simulink model "quadcopter_hadi"  (R2020a)
settings: Solver=FixedStepAuto  StartTime=0.0  StopTime=options.T_train  FixedStep=options.dt  RelTol=1e-3
undefined symbols (not defined in the file or in its folder): options
libraries: neural x134, simulink x3
(part 2 of 6)

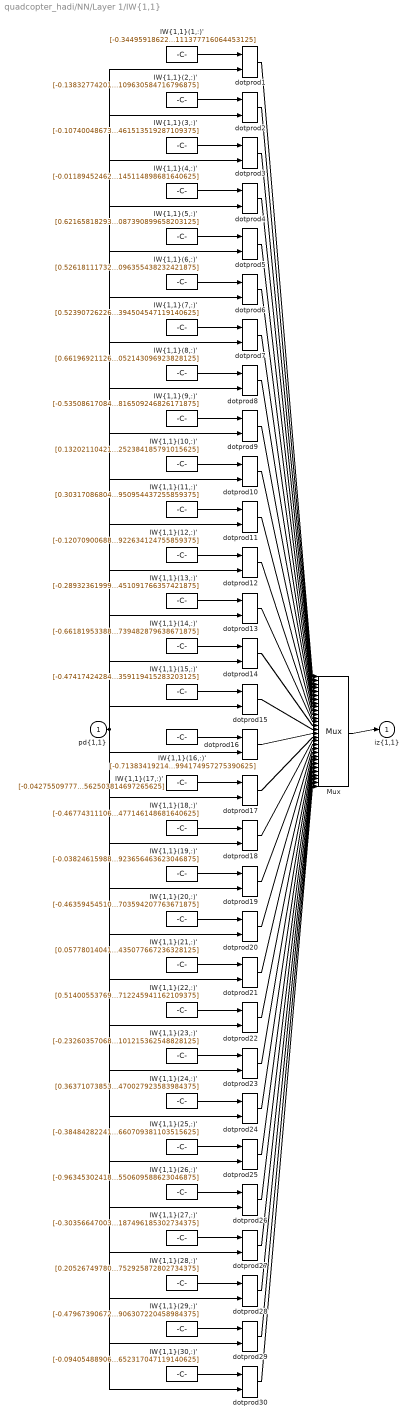
== system quadcopter_hadi/NN/Layer 1/IW{1,1} ==
  "pd{1,1}" : Inport  PortDimensions=12
      mask Display: e = 0.06;c1 = [120 230 180]/255;c2 = ([120 230 180]+0)/(256+128);c3 = ([120 230 180]+128)/(256+128);patch([0 1 1 0],[0 0 1 1],c1);patch([0 1 1 1-e 1-e 0+e],[0 0 1 1-e 0+e 0+e],c2);patch([0 0 1 1-e 0+e 0+e],[0 1 1 1-e 1-e 0+e],c3);plot([0 1 1 0 0],[0 0 1 1 0]);
  "IW{1,1}(1,:)'" : Constant  Value=[-0.34495918622896504235342263200436718761920928955078125;-0.337043723826467189752520425827242434024810791015625;-0.353509203138535899046956956226495094597339630126953125;-0.203038619812965226429923859541304409503936767578125;0.6070294560030344843681859856587834656238555908203125;-0.53053426435416162210145785138593055307865142822265625;0.40549662019742005458766698211547918617725372314453125;-0.57742825274382714173526665035751648247241973876953125;-0.318931166570593116471599159922334365546703338623046875;0.062207561993730724203555126905484939925372600555419921875;0.340697979277285567523136933232308365404605865478515625;-0.4455201013994714021038134887930937111377716064453125]
      mask Display: e = 0.06;c1 = [120 150 230]/255;c2 = ([120 150 230]+0)/383;c3 = ([120 150 230]+128)/383;patch([0 1 1 0],[0 0 1 1],c1);patch([0 1 1 1-e 1-e 0+e],[0 0 1 1-e 0+e 0+e],c2);patch([0 0 1 1-e 0+e 0+e],[0 1 1 1-e 1-e 0+e],c3);plot([0 1 1 0 0],[0 0 1 1 0]);disp('Weights');
  "IW{1,1}(10,:)'" : Constant  Value=[0.1320211042100700726820150521234609186649322509765625;-0.668627746850793958088843282894231379032135009765625;0.5677864448354277282504654067452065646648406982421875;0.0876991445872624397761541104046045802533626556396484375;-0.56179042828860958902481570476084016263484954833984375;-0.348882703813149508409452437263098545372486114501953125;0.20436817069308166328056586280581541359424591064453125;0.52533055189570043719271552618010900914669036865234375;0.9640955257051808668933290391578339040279388427734375;0.24519760024947567789155300488346256315708160400390625;-0.54886720284928236512911325917229987680912017822265625;0.257390461906887024756684922977001406252384185791015625]
      mask Display: e = 0.06;c1 = [120 150 230]/255;c2 = ([120 150 230]+0)/383;c3 = ([120 150 230]+128)/383;patch([0 1 1 0],[0 0 1 1],c1);patch([0 1 1 1-e 1-e 0+e],[0 0 1 1-e 0+e 0+e],c2);patch([0 0 1 1-e 0+e 0+e],[0 1 1 1-e 1-e 0+e],c3);plot([0 1 1 0 0],[0 0 1 1 0]);disp('Weights');
  "IW{1,1}(11,:)'" : Constant  Value=[0.303170868046250541194552852175547741353511810302734375;0.417696798526436541276751768236863426864147186279296875;0.298261926050533421328481153977918438613414764404296875;0.255036537942097740749858303388464264571666717529296875;-0.7244894696039654302666122021037153899669647216796875;0.384577235401244943435727918767952360212802886962890625;0.50089881261622692942836465590517036616802215576171875;0.309950678139630564356110653534415178000926971435546875;-0.237501763203682936254068636117153801023960113525390625;0.352274481786692350571144061177619732916355133056640625;0.416167732301852222320803775801323354244232177734375;0.319139822380907600685162606168887577950954437255859375]
      mask Display: e = 0.06;c1 = [120 150 230]/255;c2 = ([120 150 230]+0)/383;c3 = ([120 150 230]+128)/383;patch([0 1 1 0],[0 0 1 1],c1);patch([0 1 1 1-e 1-e 0+e],[0 0 1 1-e 0+e 0+e],c2);patch([0 0 1 1-e 0+e 0+e],[0 1 1 1-e 1-e 0+e],c3);plot([0 1 1 0 0],[0 0 1 1 0]);disp('Weights');
  "IW{1,1}(12,:)'" : Constant  Value=[-0.12070900688584484949927855268470011651515960693359375;0.53505476241080895949409068634849973022937774658203125;-0.2381029444773878067653782863999367691576480865478515625;-0.5429788112757945039987816926441155374050140380859375;-0.63257154591633291129681992970290593802928924560546875;-0.661157862985402022815151212853379547595977783203125;-0.60701795231436894706433804458356462419033050537109375;-0.1298953163042863290232986628325306810438632965087890625;0.84804820628712374031010767794214189052581787109375;0.126838248292744426581890593297430314123630523681640625;-0.1101413285813153120074048274545930325984954833984375;0.29384196869861722856143160242936573922634124755859375]
      mask Display: e = 0.06;c1 = [120 150 230]/255;c2 = ([120 150 230]+0)/383;c3 = ([120 150 230]+128)/383;patch([0 1 1 0],[0 0 1 1],c1);patch([0 1 1 1-e 1-e 0+e],[0 0 1 1-e 0+e 0+e],c2);patch([0 0 1 1-e 0+e 0+e],[0 1 1 1-e 1-e 0+e],c3);plot([0 1 1 0 0],[0 0 1 1 0]);disp('Weights');
  "IW{1,1}(13,:)'" : Constant  Value=[-0.289323619993917702242214318175683729350566864013671875;-0.5661963662077675873973703346564434468746185302734375;-0.263001047924680708689493258134461939334869384765625;0.763890200972800581524779772735200822353363037109375;0.58754737292300973638958794253994710743427276611328125;0.60801383959154453595630229756352491676807403564453125;-0.5265003431597750083170694779255427420139312744140625;0.1137610485372035629136888701395946554839611053466796875;-0.5072867886078873400634847712353803217411041259765625;0.469464342242350340939083253033459186553955078125;0.277240104279838639467214989053900353610515594482421875;-0.793994998950516173152891497011296451091766357421875]
      mask Display: e = 0.06;c1 = [120 150 230]/255;c2 = ([120 150 230]+0)/383;c3 = ([120 150 230]+128)/383;patch([0 1 1 0],[0 0 1 1],c1);patch([0 1 1 1-e 1-e 0+e],[0 0 1 1-e 0+e 0+e],c2);patch([0 0 1 1-e 0+e 0+e],[0 1 1 1-e 1-e 0+e],c3);plot([0 1 1 0 0],[0 0 1 1 0]);disp('Weights');
  "IW{1,1}(14,:)'" : Constant  Value=[-0.66181953388010417160813858572510071098804473876953125;-0.0703899958783368584480655272272997535765171051025390625;-0.5991581448220273387050838209688663482666015625;0.3699087288651252691806803341023623943328857421875;-0.317569978247375761526427595526911318302154541015625;0.52610263318384575814690151673858053982257843017578125;-0.27980528750779820601479741526418365538120269775390625;0.416857080760284326448328329206560738384723663330078125;0.725583975883678622409433955908752977848052978515625;0.435054608829613831399996115578687749803066253662109375;-0.458054194167220318778532828218885697424411773681640625;-0.69641998097306412329743352529476396739482879638671875]
      mask Display: e = 0.06;c1 = [120 150 230]/255;c2 = ([120 150 230]+0)/383;c3 = ([120 150 230]+128)/383;patch([0 1 1 0],[0 0 1 1],c1);patch([0 1 1 1-e 1-e 0+e],[0 0 1 1-e 0+e 0+e],c2);patch([0 0 1 1-e 0+e 0+e],[0 1 1 1-e 1-e 0+e],c3);plot([0 1 1 0 0],[0 0 1 1 0]);disp('Weights');
  "IW{1,1}(15,:)'" : Constant  Value=[-0.474174242849191351911741776348208077251911163330078125;-0.04891747802004135781128724147492903284728527069091796875;0.411091414463095439213446979920263402163982391357421875;-0.03650572612073470224469673439671169035136699676513671875;0.9444343014165463845444037360721267759799957275390625;0.59688073236543626176597854282590560615062713623046875;0.218856619672374519414148608120740391314029693603515625;0.051222945628977611942644898590515367686748504638671875;-0.53026532302764384230187033608672209084033966064453125;-0.25745047520204378255215260651311837136745452880859375;-0.28207174996604778005604430290986783802509307861328125;-0.69241459640721547685870973509736359119415283203125]
      mask Display: e = 0.06;c1 = [120 150 230]/255;c2 = ([120 150 230]+0)/383;c3 = ([120 150 230]+128)/383;patch([0 1 1 0],[0 0 1 1],c1);patch([0 1 1 1-e 1-e 0+e],[0 0 1 1-e 0+e 0+e],c2);patch([0 0 1 1-e 0+e 0+e],[0 1 1 1-e 1-e 0+e],c3);plot([0 1 1 0 0],[0 0 1 1 0]);disp('Weights');
  "IW{1,1}(16,:)'" : Constant  Value=[-0.7138341921425268576939515696722082793712615966796875;0.037340534291947467815386829670387669466435909271240234375;0.54479666790288738820180469701881520450115203857421875;-0.2021602873810667555520836913274251855909824371337890625;-0.007519167787261805437071249258451643981970846652984619140625;-0.53077415040406428214936340737040154635906219482421875;-0.5226709505181668102835601530387066304683685302734375;0.723058432424417585338005665107630193233489990234375;0.57923937859777441250486162971355952322483062744140625;-0.11337543588273957251288948100409470498561859130859375;0.401730100819205071527306927237077616155147552490234375;-0.468101990603508932853316082400851882994174957275390625]
      mask Display: e = 0.06;c1 = [120 150 230]/255;c2 = ([120 150 230]+0)/383;c3 = ([120 150 230]+128)/383;patch([0 1 1 0],[0 0 1 1],c1);patch([0 1 1 1-e 1-e 0+e],[0 0 1 1-e 0+e 0+e],c2);patch([0 0 1 1-e 0+e 0+e],[0 1 1 1-e 1-e 0+e],c3);plot([0 1 1 0 0],[0 0 1 1 0]);disp('Weights');
  "IW{1,1}(17,:)'" : Constant  Value=[-0.042755097773684337669752864030670025385916233062744140625;0.756605493708306209299507827381603419780731201171875;-0.49321543387669442015663889833376742899417877197265625;-0.325875695135673992819391742159496061503887176513671875;0.74621132739286133439549075774266384541988372802734375;-0.08679338092441117591402388597998651675879955291748046875;-0.453659556696276944354195848063682205975055694580078125;-0.62366920735145792153986121775233186781406402587890625;-0.8150300553565761330077066304511390626430511474609375;0.11508615117670083216605547704602940939366817474365234375;0.50080307025032577694645397059503011405467987060546875;-0.1889869390507021851277613677666522562503814697265625]
      mask Display: e = 0.06;c1 = [120 150 230]/255;c2 = ([120 150 230]+0)/383;c3 = ([120 150 230]+128)/383;patch([0 1 1 0],[0 0 1 1],c1);patch([0 1 1 1-e 1-e 0+e],[0 0 1 1-e 0+e 0+e],c2);patch([0 0 1 1-e 0+e 0+e],[0 1 1 1-e 1-e 0+e],c3);plot([0 1 1 0 0],[0 0 1 1 0]);disp('Weights');
  "IW{1,1}(18,:)'" : Constant  Value=[-0.46774311106672594728905778538319282233715057373046875;0.6841256626066598567348364667850546538829803466796875;0.9849894355797144118724872896564193069934844970703125;-0.68550119697938216578592118821688927710056304931640625;0.330176687462999274291775009260163642466068267822265625;-0.0757421832731329514043494555153301917016506195068359375;-0.447741975939116854110721988035948015749454498291015625;0.39313879995946365841774650107254274189472198486328125;0.039471528533331634580605395967722870409488677978515625;0.02006562823856268551470094507749308831989765167236328125;-0.39311485574848881174858661324833519756793975830078125;-0.0087918173201730898114192314096726477146148681640625]
      mask Display: e = 0.06;c1 = [120 150 230]/255;c2 = ([120 150 230]+0)/383;c3 = ([120 150 230]+128)/383;patch([0 1 1 0],[0 0 1 1],c1);patch([0 1 1 1-e 1-e 0+e],[0 0 1 1-e 0+e 0+e],c2);patch([0 0 1 1-e 0+e 0+e],[0 1 1 1-e 1-e 0+e],c3);plot([0 1 1 0 0],[0 0 1 1 0]);disp('Weights');
  "IW{1,1}(19,:)'" : Constant  Value=[-0.038246159880512074769054464695727801881730556488037109375;-0.352676020543882307034522227695561014115810394287109375;0.55521428620525714592304211691953241825103759765625;-0.236763462408719538299095574984676204621791839599609375;-0.072727039559656869727177763707004487514495849609375;0.121413069532788242543830392605741508305072784423828125;-0.305176260105177010739652132542687468230724334716796875;-0.4439076777797945627668241286301054060459136962890625;-0.98313794595444570223463642832939513027667999267578125;-0.1270463796308993476014137513629975728690624237060546875;0.902189168883986258862250906531699001789093017578125;-0.1273899410450269609196283226992818526923656463623046875]
      mask Display: e = 0.06;c1 = [120 150 230]/255;c2 = ([120 150 230]+0)/383;c3 = ([120 150 230]+128)/383;patch([0 1 1 0],[0 0 1 1],c1);patch([0 1 1 1-e 1-e 0+e],[0 0 1 1-e 0+e 0+e],c2);patch([0 0 1 1-e 0+e 0+e],[0 1 1 1-e 1-e 0+e],c3);plot([0 1 1 0 0],[0 0 1 1 0]);disp('Weights');
  "IW{1,1}(2,:)'" : Constant  Value=[-0.138327742010193599497824834543280303478240966796875;-0.8821579573578286481705390542629174888134002685546875;-0.086774823339577478176209979210398159921169281005859375;0.574481836593661920886688676546327769756317138671875;-0.529761642169075397390543002984486520290374755859375;-0.10542287766760018163925138878767029382288455963134765625;-0.439906734367202567614896224768017418682575225830078125;-0.2072733028239615304944010176768642850220203399658203125;0.56108927501055705366894699182012118399143218994140625;-0.59696070904831877168561504731769673526287078857421875;0.363071184175628058898865901937824673950672149658203125;0.826574201384250084601035268860869109630584716796875]
      mask Display: e = 0.06;c1 = [120 150 230]/255;c2 = ([120 150 230]+0)/383;c3 = ([120 150 230]+128)/383;patch([0 1 1 0],[0 0 1 1],c1);patch([0 1 1 1-e 1-e 0+e],[0 0 1 1-e 0+e 0+e],c2);patch([0 0 1 1-e 0+e 0+e],[0 1 1 1-e 1-e 0+e],c3);plot([0 1 1 0 0],[0 0 1 1 0]);disp('Weights');
  "IW{1,1}(20,:)'" : Constant  Value=[-0.463594545102451238705043579102493822574615478515625;0.59859312767452277359581103155505843460559844970703125;0.60801387674530882332391001909854821860790252685546875;-0.4376213200013177040403888895525597035884857177734375;0.465343080687624366387211694018333218991756439208984375;-0.7504994595920637667774144574650563299655914306640625;0.1096976721316818281781735322510940022766590118408203125;0.73737837988444632220108587716822512447834014892578125;-0.4011595462138346501745900241076014935970306396484375;-0.4637681719671171709507007108186371624469757080078125;-0.449027218825725438211549089828622527420520782470703125;0.1021728787905504531874356644038925878703594207763671875]
      mask Display: e = 0.06;c1 = [120 150 230]/255;c2 = ([120 150 230]+0)/383;c3 = ([120 150 230]+128)/383;patch([0 1 1 0],[0 0 1 1],c1);patch([0 1 1 1-e 1-e 0+e],[0 0 1 1-e 0+e 0+e],c2);patch([0 0 1 1-e 0+e 0+e],[0 1 1 1-e 1-e 0+e],c3);plot([0 1 1 0 0],[0 0 1 1 0]);disp('Weights');
  "IW{1,1}(21,:)'" : Constant  Value=[0.057780140416524870816683545626801787875592708587646484375;0.3446971110697958362578674496035091578960418701171875;0.449399367813893835243987950889277271926403045654296875;-0.443821935475689155481404668535105884075164794921875;-0.6004000148789756519107640997390262782573699951171875;0.5221656918855515083777163454215042293071746826171875;0.7545170196760597747243082267232239246368408203125;0.6769434357346761910179111509933136403560638427734375;-0.354202449623008230883414171330514363944530487060546875;-0.6879409685100552618308711316785775125026702880859375;-0.47037002086478107987232988307368941605091094970703125;-0.036409196162681962960494530534560908563435077667236328125]
      mask Display: e = 0.06;c1 = [120 150 230]/255;c2 = ([120 150 230]+0)/383;c3 = ([120 150 230]+128)/383;patch([0 1 1 0],[0 0 1 1],c1);patch([0 1 1 1-e 1-e 0+e],[0 0 1 1-e 0+e 0+e],c2);patch([0 0 1 1-e 0+e 0+e],[0 1 1 1-e 1-e 0+e],c3);plot([0 1 1 0 0],[0 0 1 1 0]);disp('Weights');
  "IW{1,1}(22,:)'" : Constant  Value=[0.5140055376953736043788012466393411159515380859375;-0.5947686065042745440223370678722858428955078125;0.5873305202085770115871810048702172935009002685546875;-0.3123825429203936909772210128721781075000762939453125;0.53040919266754682492859274134389124810695648193359375;-0.512060005984212640584019027301110327243804931640625;-0.58357904592260589904384460169239901006221771240234375;-0.65324640661213795311823560041375458240509033203125;0.11144911224205389377317487742402590811252593994140625;0.518976412161789912858012030483223497867584228515625;0.444696308915158267094369648475549183785915374755859375;0.37402510131684285621389562948024831712245941162109375]
      mask Display: e = 0.06;c1 = [120 150 230]/255;c2 = ([120 150 230]+0)/383;c3 = ([120 150 230]+128)/383;patch([0 1 1 0],[0 0 1 1],c1);patch([0 1 1 1-e 1-e 0+e],[0 0 1 1-e 0+e 0+e],c2);patch([0 0 1 1-e 0+e 0+e],[0 1 1 1-e 1-e 0+e],c3);plot([0 1 1 0 0],[0 0 1 1 0]);disp('Weights');
  "IW{1,1}(23,:)'" : Constant  Value=[-0.232603570682247184908675308179226703941822052001953125;1.0517575952902709079950227533117868006229400634765625;0.192098506547794423138242336790426634252071380615234375;-0.32973101267621285348496940059703774750232696533203125;-0.11914062282579916673963538187308586202561855316162109375;-0.382401536887546911192004017721046693623065948486328125;-0.35312961938715103915598092498839832842350006103515625;0.164251234547107827221879006174276582896709442138671875;0.407895691716687769368121507795876823365688323974609375;-0.8752379671019092644002057568286545574665069580078125;0.413170407813726325851888532270095311105251312255859375;0.61017749365807916195336702003260143101215362548828125]
      mask Display: e = 0.06;c1 = [120 150 230]/255;c2 = ([120 150 230]+0)/383;c3 = ([120 150 230]+128)/383;patch([0 1 1 0],[0 0 1 1],c1);patch([0 1 1 1-e 1-e 0+e],[0 0 1 1-e 0+e 0+e],c2);patch([0 0 1 1-e 0+e 0+e],[0 1 1 1-e 1-e 0+e],c3);plot([0 1 1 0 0],[0 0 1 1 0]);disp('Weights');
  "IW{1,1}(24,:)'" : Constant  Value=[0.363710738539707645333720620328676886856555938720703125;-0.09612229443336224588012584035823238082230091094970703125;0.1808198562023227429218508177655166946351528167724609375;-0.4720334048143357552618226691265590488910675048828125;-0.294063177509011897114987732493318617343902587890625;0.87626234603710873027893057951587252318859100341796875;-0.634035117918139601300708818598650395870208740234375;-0.5522125975537324205077993610757403075695037841796875;-0.17623578995034094862859319619019515812397003173828125;0.43632440477811285095555149382562376558780670166015625;0.89163382673504631981131751672364771366119384765625;-0.167074453475141326830311072626500390470027923583984375]
      mask Display: e = 0.06;c1 = [120 150 230]/255;c2 = ([120 150 230]+0)/383;c3 = ([120 150 230]+128)/383;patch([0 1 1 0],[0 0 1 1],c1);patch([0 1 1 1-e 1-e 0+e],[0 0 1 1-e 0+e 0+e],c2);patch([0 0 1 1-e 0+e 0+e],[0 1 1 1-e 1-e 0+e],c3);plot([0 1 1 0 0],[0 0 1 1 0]);disp('Weights');
  "IW{1,1}(25,:)'" : Constant  Value=[-0.38484282241698941628982311158324591815471649169921875;0.209383083397630065380923269913182593882083892822265625;-0.6135781360303920184406933913123793900012969970703125;0.76016324948769209424170867350767366588115692138671875;-0.362471393437067190834710572744370438158512115478515625;-0.60581492990217078453696331052924506366252899169921875;0.585753156661642293556724325753748416900634765625;-0.50309249495567087695491181875695474445819854736328125;0.48695535648605725587145798272104002535343170166015625;0.714144675850457932853032616549171507358551025390625;-0.27025145430345942632044398123980499804019927978515625;0.541591787927542700487038018763996660709381103515625]
      mask Display: e = 0.06;c1 = [120 150 230]/255;c2 = ([120 150 230]+0)/383;c3 = ([120 150 230]+128)/383;patch([0 1 1 0],[0 0 1 1],c1);patch([0 1 1 1-e 1-e 0+e],[0 0 1 1-e 0+e 0+e],c2);patch([0 0 1 1-e 0+e 0+e],[0 1 1 1-e 1-e 0+e],c3);plot([0 1 1 0 0],[0 0 1 1 0]);disp('Weights');
  "IW{1,1}(26,:)'" : Constant  Value=[-0.96345302418685896395089685029233805835247039794921875;0.2905057488862652359529192835907451808452606201171875;0.25145319652790931730379497821559198200702667236328125;-0.110023152779389732369708099213312380015850067138671875;0.80159591366269555834378479630686342716217041015625;0.62482096118850416477386033875518478453159332275390625;0.1804782462712755941591780128874233923852443695068359375;-0.69123516144817764850216690319939516484737396240234375;-0.32694257387283298665892061762860976159572601318359375;0.04918257558373796689554779959507868625223636627197265625;-0.66886565497689642878498261779895983636379241943359375;-0.27607850951602752598290635432931594550609588623046875]
      mask Display: e = 0.06;c1 = [120 150 230]/255;c2 = ([120 150 230]+0)/383;c3 = ([120 150 230]+128)/383;patch([0 1 1 0],[0 0 1 1],c1);patch([0 1 1 1-e 1-e 0+e],[0 0 1 1-e 0+e 0+e],c2);patch([0 0 1 1-e 0+e 0+e],[0 1 1 1-e 1-e 0+e],c3);plot([0 1 1 0 0],[0 0 1 1 0]);disp('Weights');
  "IW{1,1}(27,:)'" : Constant  Value=[-0.30356647003768255643763041007332503795623779296875;0.397535672113617177814148817560635507106781005859375;-0.12467461340805656433428083573744515888392925262451171875;-0.70752774859209655033964736503548920154571533203125;0.66465656668955952479649340602918528020381927490234375;-0.034394405255799960496876366278229397721588611602783203125;0.48028770547293431203428326625726185739040374755859375;-0.54949688236805938057472076252452097833156585693359375;-0.81716499127206809749424110123072750866413116455078125;-0.00698809762742241304123158585070996196009218692779541015625;0.66303543817856114284126078928238712251186370849609375;0.126087445960947286405229306183173321187496185302734375]
      mask Display: e = 0.06;c1 = [120 150 230]/255;c2 = ([120 150 230]+0)/383;c3 = ([120 150 230]+128)/383;patch([0 1 1 0],[0 0 1 1],c1);patch([0 1 1 1-e 1-e 0+e],[0 0 1 1-e 0+e 0+e],c2);patch([0 0 1 1-e 0+e 0+e],[0 1 1 1-e 1-e 0+e],c3);plot([0 1 1 0 0],[0 0 1 1 0]);disp('Weights');
  "IW{1,1}(28,:)'" : Constant  Value=[0.2052674978043443621000818666288978420197963714599609375;0.35070641269276559004453019952052272856235504150390625;0.63836983163101723715016078131156973540782928466796875;0.391881550618063290158943345886655151844024658203125;-0.171565904611522268563561510745785199105739593505859375;-0.54250734055331950589362577375140972435474395751953125;-0.70606196712206215071461201659985817968845367431640625;0.315078701273152239625829906799481250345706939697265625;0.7571027888427377394719997028005309402942657470703125;0.374860392792828178709640951637993566691875457763671875;-0.2434391219306188958171333069913089275360107421875;0.44060900182772877453629689625813625752925872802734375]
      mask Display: e = 0.06;c1 = [120 150 230]/255;c2 = ([120 150 230]+0)/383;c3 = ([120 150 230]+128)/383;patch([0 1 1 0],[0 0 1 1],c1);patch([0 1 1 1-e 1-e 0+e],[0 0 1 1-e 0+e 0+e],c2);patch([0 0 1 1-e 0+e 0+e],[0 1 1 1-e 1-e 0+e],c3);plot([0 1 1 0 0],[0 0 1 1 0]);disp('Weights');
  "IW{1,1}(29,:)'" : Constant  Value=[-0.47967390672573750887153209987445734441280364990234375;-0.1710937102409248178336298451540642417967319488525390625;0.51569510317060884840856260780128650367259979248046875;0.58303215536935770746396201502648182213306427001953125;0.5397101537550013095057011014432646334171295166015625;0.491815641277797033215080091395066119730472564697265625;-0.26359399694002305647444472924689762294292449951171875;-0.5159654272192575330535646571661345660686492919921875;-0.795397536289371931417235828121192753314971923828125;-0.67850322234585813685470156997325830161571502685546875;0.394304169753736000192390065421932376921176910400390625;0.08171990282033135544192958832354634068906307220458984375]
      mask Display: e = 0.06;c1 = [120 150 230]/255;c2 = ([120 150 230]+0)/383;c3 = ([120 150 230]+128)/383;patch([0 1 1 0],[0 0 1 1],c1);patch([0 1 1 1-e 1-e 0+e],[0 0 1 1-e 0+e 0+e],c2);patch([0 0 1 1-e 0+e 0+e],[0 1 1 1-e 1-e 0+e],c3);plot([0 1 1 0 0],[0 0 1 1 0]);disp('Weights');
  "IW{1,1}(3,:)'" : Constant  Value=[-0.10740048673439391013761934345893678255379199981689453125;-0.2172720702613431253968911960328114219009876251220703125;0.2378394016623203988114454432434285990893840789794921875;0.51394110379334267957318616026896052062511444091796875;0.37661624669478188653926054030307568609714508056640625;0.487273539589460569221301966535975225269794464111328125;0.42566721914787331026985839343979023396968841552734375;-0.8937639297673716232139895510044880211353302001953125;-0.135569594033347284867119242335320450365543365478515625;0.8757068982107643062562374325352720916271209716796875;0.361943270803529892898353637065156362950801849365234375;-0.135562992761426581722616901970468461513519287109375]
      mask Display: e = 0.06;c1 = [120 150 230]/255;c2 = ([120 150 230]+0)/383;c3 = ([120 150 230]+128)/383;patch([0 1 1 0],[0 0 1 1],c1);patch([0 1 1 1-e 1-e 0+e],[0 0 1 1-e 0+e 0+e],c2);patch([0 0 1 1-e 0+e 0+e],[0 1 1 1-e 1-e 0+e],c3);plot([0 1 1 0 0],[0 0 1 1 0]);disp('Weights');
  "IW{1,1}(30,:)'" : Constant  Value=[-0.09405488906321969599932941719089285470545291900634765625;-0.467610333580071202419503606506623327732086181640625;-0.159695215182861172120709625232848338782787322998046875;0.322947655372797848283283883574767969548702239990234375;0.337291546166701483588923338174936361610889434814453125;-0.5604847262703398502736718000960536301136016845703125;-0.51864010655251202575044544573756866157054901123046875;0.55916502354967179133637955601443536579608917236328125;-0.379802758147711305714011587042477913200855255126953125;0.91760468236122061380655168250086717307567596435546875;-0.04817922357743227579351952272190828807651996612548828125;-0.79844520344081149065829094979562796652317047119140625]
      mask Display: e = 0.06;c1 = [120 150 230]/255;c2 = ([120 150 230]+0)/383;c3 = ([120 150 230]+128)/383;patch([0 1 1 0],[0 0 1 1],c1);patch([0 1 1 1-e 1-e 0+e],[0 0 1 1-e 0+e 0+e],c2);patch([0 0 1 1-e 0+e 0+e],[0 1 1 1-e 1-e 0+e],c3);plot([0 1 1 0 0],[0 0 1 1 0]);disp('Weights');
  "IW{1,1}(4,:)'" : Constant  Value=[-0.01189452462799470318366434895551719819195568561553955078125;0.30955222784386149381674613323411904275417327880859375;0.37405694379270337801557388957007788121700286865234375;-0.337930186454908021431720044347457587718963623046875;0.5586613099046164876426701084710657596588134765625;0.66911143805661854599975413293577730655670166015625;-0.71804193868486254626049003491061739623546600341796875;-0.30199328076909093265811634410056285560131072998046875;0.479407886897864343733743908160249702632427215576171875;-0.2214060732027794686782584676620899699628353118896484375;-0.52388837611547189876404218011884950101375579833984375;0.9040601619831820645600828356691636145114898681640625]
      mask Display: e = 0.06;c1 = [120 150 230]/255;c2 = ([120 150 230]+0)/383;c3 = ([120 150 230]+128)/383;patch([0 1 1 0],[0 0 1 1],c1);patch([0 1 1 1-e 1-e 0+e],[0 0 1 1-e 0+e 0+e],c2);patch([0 0 1 1-e 0+e 0+e],[0 1 1 1-e 1-e 0+e],c3);plot([0 1 1 0 0],[0 0 1 1 0]);disp('Weights');
  "IW{1,1}(5,:)'" : Constant  Value=[0.62165818293616614820251697892672382295131683349609375;0.397865582455294575225934750051237642765045166015625;0.7316722067555614383849160731188021600246429443359375;-0.487716561673313453439959630486555397510528564453125;-0.30403759874493208048562564727035351097583770751953125;0.36844925044632315103143582746270112693309783935546875;-0.2266763489839582756957270248676650226116180419921875;-0.332136918694305782739917276558117009699344635009765625;0.1219087873483228889881502254866063594818115234375;0.48112981175821623036625851455028168857097625732421875;0.3560647281492952398451734552509151399135589599609375;0.55496834794659843925757058968883939087390899658203125]
      mask Display: e = 0.06;c1 = [120 150 230]/255;c2 = ([120 150 230]+0)/383;c3 = ([120 150 230]+128)/383;patch([0 1 1 0],[0 0 1 1],c1);patch([0 1 1 1-e 1-e 0+e],[0 0 1 1-e 0+e 0+e],c2);patch([0 0 1 1-e 0+e 0+e],[0 1 1 1-e 1-e 0+e],c3);plot([0 1 1 0 0],[0 0 1 1 0]);disp('Weights');
  "IW{1,1}(6,:)'" : Constant  Value=[0.52618111732526784418695342537830583751201629638671875;-0.440625471004194635415984748760820366442203521728515625;-0.62487389944786653206421078721177764236927032470703125;-0.0222850483937825256941511753439044696278870105743408203125;0.5691934711227240040187780323321931064128875732421875;-0.90291982242941315472961605337332002818584442138671875;0.417050626719000394615477489423938095569610595703125;-0.177028368010524517206505379363079555332660675048828125;-0.15451508861587426313377591213793493807315826416015625;0.75850356023963472207327640717267058789730072021484375;-0.195424851993045878284505079136579297482967376708984375;0.1381647165547894295922759511086042039096355438232421875]
      mask Display: e = 0.06;c1 = [120 150 230]/255;c2 = ([120 150 230]+0)/383;c3 = ([120 150 230]+128)/383;patch([0 1 1 0],[0 0 1 1],c1);patch([0 1 1 1-e 1-e 0+e],[0 0 1 1-e 0+e 0+e],c2);patch([0 0 1 1-e 0+e 0+e],[0 1 1 1-e 1-e 0+e],c3);plot([0 1 1 0 0],[0 0 1 1 0]);disp('Weights');
  "IW{1,1}(7,:)'" : Constant  Value=[0.5239072622656049116329768366995267570018768310546875;-0.3432914261529236288339461680152453482151031494140625;-0.7086167696794871684318195548257790505886077880859375;0.5572090256839017374801414916873909533023834228515625;-0.56712716940789198449834884740994311869144439697265625;0.061168833619787581212801086394392768852412700653076171875;-0.643665616440932009112430023378692567348480224609375;-0.38315560147590821404861571863875724375247955322265625;0.52732661808370517864119619844132103025913238525390625;0.4970608747190905507551406117272563278675079345703125;0.224618568925987471818217500185710377991199493408203125;-0.344126400018276046299803283545770682394504547119140625]
      mask Display: e = 0.06;c1 = [120 150 230]/255;c2 = ([120 150 230]+0)/383;c3 = ([120 150 230]+128)/383;patch([0 1 1 0],[0 0 1 1],c1);patch([0 1 1 1-e 1-e 0+e],[0 0 1 1-e 0+e 0+e],c2);patch([0 0 1 1-e 0+e 0+e],[0 1 1 1-e 1-e 0+e],c3);plot([0 1 1 0 0],[0 0 1 1 0]);disp('Weights');
  "IW{1,1}(8,:)'" : Constant  Value=[0.661969211261337786567082730471156537532806396484375;-0.0383159852429298675158264586571021936833858489990234375;-0.09722917799189277621163540743509656749665737152099609375;0.2607808122246872972738174212281592190265655517578125;-0.89249206258839197669630038944887928664684295654296875;0.290074660908613335408290367922745645046234130859375;0.082028400526420741645239331774064339697360992431640625;0.52493892311090950553165157543844543397426605224609375;0.76704115696658570211496908086701296269893646240234375;-0.240414255138845456283291923682554624974727630615234375;-0.023871623658473208051677971752724261023104190826416015625;-0.63902701740953304909709231651504524052143096923828125]
      mask Display: e = 0.06;c1 = [120 150 230]/255;c2 = ([120 150 230]+0)/383;c3 = ([120 150 230]+128)/383;patch([0 1 1 0],[0 0 1 1],c1);patch([0 1 1 1-e 1-e 0+e],[0 0 1 1-e 0+e 0+e],c2);patch([0 0 1 1-e 0+e 0+e],[0 1 1 1-e 1-e 0+e],c3);plot([0 1 1 0 0],[0 0 1 1 0]);disp('Weights');
  "IW{1,1}(9,:)'" : Constant  Value=[-0.53508617084060328128458650098764337599277496337890625;0.0795815485999021021701338440834661014378070831298828125;-0.66131439300399819103404297493398189544677734375;0.198887915850595120570432072781841270625591278076171875;-0.4638113422795602236448075927910394966602325439453125;-0.5485711737735516901892651731031946837902069091796875;0.39899541815562844515596907513099722564220428466796875;-0.017703826639693880096171341165245394222438335418701171875;0.91695552187400952703910661512054502964019775390625;-0.148963777410568931625078903380199335515499114990234375;-0.43559264363035443690108650116599164903163909912109375;-0.27085804944175506658865515419165603816509246826171875]
      mask Display: e = 0.06;c1 = [120 150 230]/255;c2 = ([120 150 230]+0)/383;c3 = ([120 150 230]+128)/383;patch([0 1 1 0],[0 0 1 1],c1);patch([0 1 1 1-e 1-e 0+e],[0 0 1 1-e 0+e 0+e],c2);patch([0 0 1 1-e 0+e 0+e],[0 1 1 1-e 1-e 0+e],c3);plot([0 1 1 0 0],[0 0 1 1 0]);disp('Weights');
  Mux : Mux  Inputs=30
      mask Display: e = 0.06;c1 = [120 150 230]/255;c2 = ([120 150 230]+0)/383;c3 = ([120 150 230]+128)/383;patch([0 1 1 0],[0 0 1 1],c1);patch([0 1 1 1-e 1-e 0+e],[0 0 1 1-e 0+e 0+e],c2);patch([0 0 1 1-e 0+e 0+e],[0 1 1 1-e 1-e 0+e],c3);plot([0 1 1 0 0],[0 0 1 1 0]);disp('Mux');
  dotprod{1..30} (30 alike) : neural/Weight Functions/dotprod
  "iz{1,1}" : Outport
      mask Display: e = 0.06;c1 = [120 230 180]/255;c2 = ([120 230 180]+0)/(256+128);c3 = ([120 230 180]+128)/(256+128);patch([0 1 1 0],[0 0 1 1],c1);patch([0 1 1 1-e 1-e 0+e],[0 0 1 1-e 0+e 0+e],c2);patch([0 0 1 1-e 0+e 0+e],[0 1 1 1-e 1-e 0+e],c3);plot([0 1 1 0 0],[0 0 1 1 0]);
  wires:
  "IW{1,1}(1,:)'"/1 -> dotprod1/1
  "pd{1,1}"/1 -> dotprod1/2, dotprod2/2, dotprod3/2, dotprod4/2, dotprod5/2, dotprod6/2, dotprod7/2, dotprod8/2, dotprod9/2, dotprod10/2, dotprod11/2, dotprod12/2, dotprod13/2, dotprod14/2, dotprod15/2, dotprod16/2, dotprod17/2, dotprod18/2, dotprod19/2, dotprod20/2, dotprod21/2, dotprod22/2, dotprod23/2, dotprod24/2, dotprod25/2, dotprod26/2, dotprod27/2, dotprod28/2, dotprod29/2, dotprod30/2
  dotprod1/1 -> Mux/1
  "IW{1,1}(2,:)'"/1 -> dotprod2/1
  dotprod2/1 -> Mux/2
  "IW{1,1}(3,:)'"/1 -> dotprod3/1
  dotprod3/1 -> Mux/3
  "IW{1,1}(4,:)'"/1 -> dotprod4/1
  dotprod4/1 -> Mux/4
  "IW{1,1}(5,:)'"/1 -> dotprod5/1
  dotprod5/1 -> Mux/5
  "IW{1,1}(6,:)'"/1 -> dotprod6/1
  dotprod6/1 -> Mux/6
  "IW{1,1}(7,:)'"/1 -> dotprod7/1
  dotprod7/1 -> Mux/7
  "IW{1,1}(8,:)'"/1 -> dotprod8/1
  dotprod8/1 -> Mux/8
  "IW{1,1}(9,:)'"/1 -> dotprod9/1
  dotprod9/1 -> Mux/9
  "IW{1,1}(10,:)'"/1 -> dotprod10/1
  dotprod10/1 -> Mux/10
  "IW{1,1}(11,:)'"/1 -> dotprod11/1
  dotprod11/1 -> Mux/11
  "IW{1,1}(12,:)'"/1 -> dotprod12/1
  dotprod12/1 -> Mux/12
  "IW{1,1}(13,:)'"/1 -> dotprod13/1
  dotprod13/1 -> Mux/13
  "IW{1,1}(14,:)'"/1 -> dotprod14/1
  dotprod14/1 -> Mux/14
  "IW{1,1}(15,:)'"/1 -> dotprod15/1
  dotprod15/1 -> Mux/15
  "IW{1,1}(16,:)'"/1 -> dotprod16/1
  dotprod16/1 -> Mux/16
  "IW{1,1}(17,:)'"/1 -> dotprod17/1
  dotprod17/1 -> Mux/17
  "IW{1,1}(18,:)'"/1 -> dotprod18/1
  dotprod18/1 -> Mux/18
  "IW{1,1}(19,:)'"/1 -> dotprod19/1
  dotprod19/1 -> Mux/19
  "IW{1,1}(20,:)'"/1 -> dotprod20/1
  dotprod20/1 -> Mux/20
  "IW{1,1}(21,:)'"/1 -> dotprod21/1
  dotprod21/1 -> Mux/21
  "IW{1,1}(22,:)'"/1 -> dotprod22/1
  dotprod22/1 -> Mux/22
  "IW{1,1}(23,:)'"/1 -> dotprod23/1
  dotprod23/1 -> Mux/23
  "IW{1,1}(24,:)'"/1 -> dotprod24/1
  dotprod24/1 -> Mux/24
  "IW{1,1}(25,:)'"/1 -> dotprod25/1
  dotprod25/1 -> Mux/25
  "IW{1,1}(26,:)'"/1 -> dotprod26/1
  dotprod26/1 -> Mux/26
  "IW{1,1}(27,:)'"/1 -> dotprod27/1
  dotprod27/1 -> Mux/27
  "IW{1,1}(28,:)'"/1 -> dotprod28/1
  dotprod28/1 -> Mux/28
  "IW{1,1}(29,:)'"/1 -> dotprod29/1
  dotprod29/1 -> Mux/29
  "IW{1,1}(30,:)'"/1 -> dotprod30/1
  dotprod30/1 -> Mux/30
  Mux/1 -> "iz{1,1}"/1

== system quadcopter_hadi/NN/Layer 2/Delays 1 ==
  "p{2}" : Inport  PortDimensions=30
      mask Display: e = 0.06;c1 = [120 230 180]/255;c2 = ([120 230 180]+0)/(256+128);c3 = ([120 230 180]+128)/(256+128);patch([0 1 1 0],[0 0 1 1],c1);patch([0 1 1 1-e 1-e 0+e],[0 0 1 1-e 0+e 0+e],c2);patch([0 0 1 1-e 0+e 0+e],[0 1 1 1-e 1-e 0+e],c3);plot([0 1 1 0 0],[0 0 1 1 0]);
  mux : Mux  Inputs=1
      mask Display: e = 0.06;c1 = [120 150 230]/255;c2 = ([120 150 230]+0)/383;c3 = ([120 150 230]+128)/383;patch([0 1 1 0],[0 0 1 1],c1);patch([0 1 1 1-e 1-e 0+e],[0 0 1 1-e 0+e 0+e],c2);patch([0 0 1 1-e 0+e 0+e],[0 1 1 1-e 1-e 0+e],c3);plot([0 1 1 0 0],[0 0 1 1 0]);disp('Mux')
  "pd{2,1}" : Outport
      mask Display: e = 0.06;c1 = [120 230 180]/255;c2 = ([120 230 180]+0)/(256+128);c3 = ([120 230 180]+128)/(256+128);patch([0 1 1 0],[0 0 1 1],c1);patch([0 1 1 1-e 1-e 0+e],[0 0 1 1-e 0+e 0+e],c2);patch([0 0 1 1-e 0+e 0+e],[0 1 1 1-e 1-e 0+e],c3);plot([0 1 1 0 0],[0 0 1 1 0]);
  wires:
  "p{2}"/1 -> mux/1
  mux/1 -> "pd{2,1}"/1
